simulink model "regobs"  (Simulink 2.20)
settings: Solver=ode45  StartTime=0.0  StopTime=ftime  RelTol=1e-3  AbsTol=1e-6
values from neighbouring files (symbols this model uses):
  A = [-den(2:N)' eye(N-1,N-2)]    [abodep.m]    (also in anyq.m; bodep.m; demo1.m = [0 1 0 0;23.1 0 0 -.11892627;0 0 0 1; 0 0 0 -25]; demo2.m = [      0         0         0    1.0000)
  b = p' * b    [abodep.m]    (also in anyq.m; bodep.m; demo1.m = [0;12.5253;0;2633]; demo2.m = [         0         0         0)
  c = c * p    [abodep.m]    (also in anyq.m; bodep.m; demo2.m = [ 1.0000         0         0         0; fbg.m = cond([Xt X2]))
  K = K'    [roo.m]
  L = R\B'*Y/X    [alqfbg.m]    (also in anyq.m = [L(1:npoints) d L(npoints+1:2*npoints)]; ats.m = fbg(phid,gammad,sroots2); demo1.m = fbg(phi,gamma,exp(T*s4/0.95)); dts.m = fbg(phid,gammad,zroots2))
  T = c    [bodep.m]    (also in demo1.m = 0.01; demo2.m = 0.02; fbg.m = null([(p(i)*I-A) B]))
  x0 = [0;.1;0;0]    [demo1.m]    (also in demo2.m = [0 0 0 0]')
undefined symbols (not defined in the file or in its folder): gamma, phi
settings Model: TimeSaveName=t  SaveState=on  ConsistencyChecking=off  RTWPlaceOutputsASAP=off

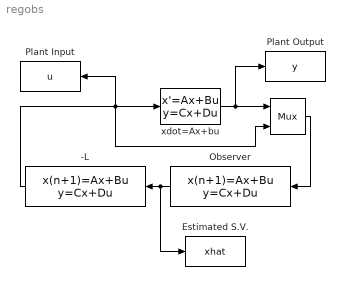
== system regobs ==
  " " : Mux  Inputs=2
  -L : DiscreteStateSpace  Orientation=left  A=0  B=zeros(1,length(A))  C=0  D=-L  X0=0  SampleTime=T
  Estimated S.V. : ToWorkspace  VariableName=xhat  SampleTime=-1
  Observer : DiscreteStateSpace  Orientation=left  A=phi-K*c  B=[K gamma]  C=eye(length(phi))  D=zeros(length(A),sum(size(c))+sum(size(b))-2*length(A))  X0=c'/(c*c')*c*x0  SampleTime=T
  Plant Input : ToWorkspace  VariableName=u  SampleTime=-1
  Plant Output : ToWorkspace  VariableName=y  SampleTime=-1
  xdot=Ax+bu : StateSpace  A=A  B=b  C=c  D=zeros(sum(size(c))-length(A),sum(size(b))-length(A))  X0=x0
  wires:
  -L/1 -> xdot=Ax+bu/1, Plant Input/1, " "/2
  " "/1 -> Observer/1
  xdot=Ax+bu/1 -> " "/1, Plant Output/1
  Observer/1 -> -L/1, Estimated S.V./1
